simulink model "scanner_design_3d"  (R2023a)
settings: Solver=VariableStepAuto  StartTime=0.0  StopTime=10.0  RelTol=1e-3
settings Model: Creator=lenovo  LastModifiedBy=lenovo

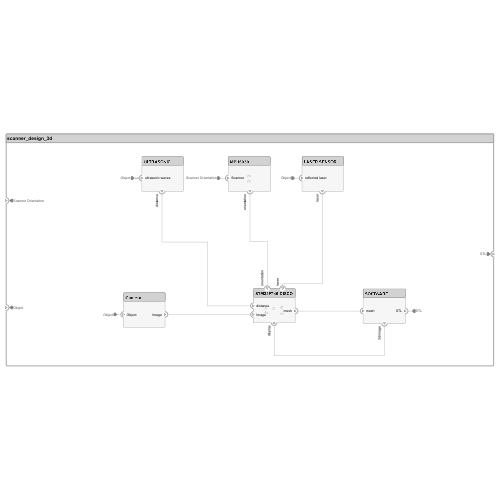
[thumbnail: Simulink's stored preview of the top-level diagram]
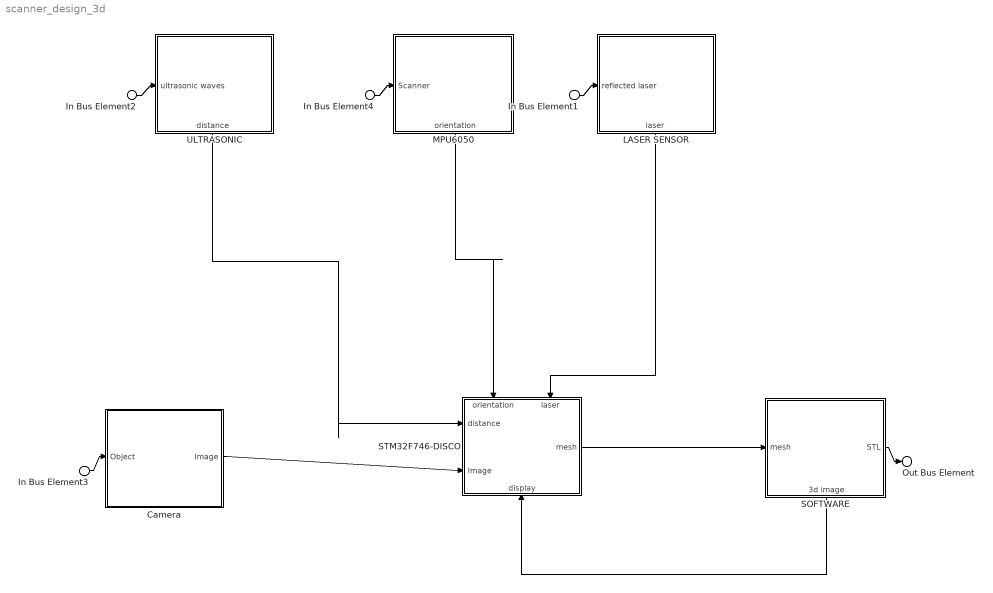
== system scanner_design_3d ==
  In Bus Element4 : Inport  PortName=Scanner Orientation
  In Bus Element1 : Inport  Port=2  PortName=Object
  In Bus Element3 : Inport  Port=2  PortName=Object
  In Bus Element2 : Inport  Port=2  PortName=Object
  Camera : Subsystem
      settings: PortSchema="{\"entries\":[{\"content\":{\"headerSize\":26,\"margin\":15,\"minimumSpacing\":25,\"sides\":[{\"content\":{\"connectorIds\":[\"In1\"]},\"type\":\"ConnectorPlacement.EquallySpacedRectSide\",\"uuid\":\"2eee4fd0-a715-4275-a226-480a0d6abb5e\"},{\"content\":{\"connectorIds\":[\"Out1\"],\"side\":\"RIGHT\"},\"type\":\"ConnectorPlacement.EquallySpacedRectSide\",\"uuid\":\"cdef6956-26e3-4994-be7c-9f37706eab71\"},{\"content\":{\"side\":\"TOP\"},\"type\":\"ConnectorPlacement.EquallySpacedRectSide\",\"uuid\":\"d49d9082-8e39-4dea-9a4e-805e3e59c1db\"}]},\"type\":\"ConnectorPlacement.EquallySpacedConnector\",\"uuid\":\"d2393f48-2e3c-4715-90d2-b77770385fe3\"}],\"packageUris\":[\"http://schema.mathworks.com/mf0/Connector/R2020b\"],\"version\":\"1.0\"}"
  LASER SENSOR : Subsystem
      settings: PortSchema="{\"entries\":[{\"content\":{\"headerSize\":26,\"margin\":15,\"minimumSpacing\":25,\"sides\":[{\"content\":{\"connectorIds\":[\"In1\"]},\"type\":\"ConnectorPlacement.EquallySpacedRectSide\",\"uuid\":\"2eee4fd0-a715-4275-a226-480a0d6abb5e\"},{\"content\":{\"side\":\"RIGHT\"},\"type\":\"ConnectorPlacement.EquallySpacedRectSide\",\"uuid\":\"cdef6956-26e3-4994-be7c-9f37706eab71\"},{\"content\":{\"side\":\"TOP\"},\"type\":\"ConnectorPlacement.EquallySpacedRectSide\",\"uuid\":\"d49d9082-8e39-4dea-9a4e-805e3e59c1db\"},{\"content\":{\"connectorIds\":[\"Out1\"],\"side\":\"BOTTOM\"},\"type\":\"ConnectorPlacement.EquallySpacedRectSide\",\"uuid\":\"d8085a13-85a2-42d5-92f1-ff20fd15cc84\"}]},\"type\":\"ConnectorPlacement.EquallySpacedConnector\",\"uuid\":\"d2393f48-2e3c-4715-90d2-b77770385fe3\"}],\"packageUris\":[\"http://schema.mathworks.com/mf0/Connector/R2020b\"],\"version\":\"1.0\"}"
  MPU6050 : Subsystem
      settings: PortSchema="{\"entries\":[{\"content\":{\"headerSize\":26,\"margin\":15,\"minimumSpacing\":25,\"sides\":[{\"content\":{\"connectorIds\":[\"In1\"]},\"type\":\"ConnectorPlacement.EquallySpacedRectSide\",\"uuid\":\"2eee4fd0-a715-4275-a226-480a0d6abb5e\"},{\"content\":{\"side\":\"RIGHT\"},\"type\":\"ConnectorPlacement.EquallySpacedRectSide\",\"uuid\":\"cdef6956-26e3-4994-be7c-9f37706eab71\"},{\"content\":{\"side\":\"TOP\"},\"type\":\"ConnectorPlacement.EquallySpacedRectSide\",\"uuid\":\"d49d9082-8e39-4dea-9a4e-805e3e59c1db\"},{\"content\":{\"connectorIds\":[\"Out1\"],\"side\":\"BOTTOM\"},\"type\":\"ConnectorPlacement.EquallySpacedRectSide\",\"uuid\":\"b078de67-0ec8-4653-9c4d-612ceac8148a\"}]},\"type\":\"ConnectorPlacement.EquallySpacedConnector\",\"uuid\":\"d2393f48-2e3c-4715-90d2-b77770385fe3\"}],\"packageUris\":[\"http://schema.mathworks.com/mf0/Connector/R2020b\"],\"version\":\"1.0\"}"
  SOFTWARE : Subsystem
      settings: PortSchema="{\"entries\":[{\"content\":{\"headerSize\":26,\"margin\":15,\"minimumSpacing\":25,\"sides\":[{\"content\":{\"connectorIds\":[\"In1\"]},\"type\":\"ConnectorPlacement.EquallySpacedRectSide\",\"uuid\":\"2eee4fd0-a715-4275-a226-480a0d6abb5e\"},{\"content\":{\"connectorIds\":[\"Out1\"],\"side\":\"RIGHT\"},\"type\":\"ConnectorPlacement.EquallySpacedRectSide\",\"uuid\":\"cdef6956-26e3-4994-be7c-9f37706eab71\"},{\"content\":{\"side\":\"TOP\"},\"type\":\"ConnectorPlacement.EquallySpacedRectSide\",\"uuid\":\"d49d9082-8e39-4dea-9a4e-805e3e59c1db\"},{\"content\":{\"connectorIds\":[\"Out2\"],\"side\":\"BOTTOM\"},\"type\":\"ConnectorPlacement.EquallySpacedRectSide\",\"uuid\":\"0b6c6432-b892-45d8-8b41-6b664d115c4f\"}]},\"type\":\"ConnectorPlacement.EquallySpacedConnector\",\"uuid\":\"d2393f48-2e3c-4715-90d2-b77770385fe3\"}],\"packageUris\":[\"http://schema.mathworks.com/mf0/Connector/R2020b\"],\"version\":\"1.0\"}"
  STM32F746-DISCO : Subsystem
      settings: PortSchema="{\"entries\":[{\"content\":{\"headerSize\":26,\"margin\":15,\"minimumSpacing\":25,\"sides\":[{\"content\":{\"connectorIds\":[\"In3\",\"In2\"]},\"type\":\"ConnectorPlacement.EquallySpacedRectSide\",\"uuid\":\"2eee4fd0-a715-4275-a226-480a0d6abb5e\"},{\"content\":{\"connectorIds\":[\"Out1\"],\"side\":\"RIGHT\"},\"type\":\"ConnectorPlacement.EquallySpacedRectSide\",\"uuid\":\"cdef6956-26e3-4994-be7c-9f37706eab71\"},{\"content\":{\"connectorIds\":[\"In4\",\"In5\"],\"side\":\"TOP\"},\"type\":\"ConnectorPlacement.EquallySpacedRectSide\",\"uuid\":\"d49d9082-8e39-4dea-9a4e-805e3e59c1db\"},{\"content\":{\"connectorIds\":[\"In1\"],\"side\":\"BOTTOM\"},\"type\":\"ConnectorPlacement.EquallySpacedRectSide\",\"uuid\":\"f1ce8cd9-933c-4617-8e31-b493098c4f66\"}]},\"type\":\"ConnectorPlacement.EquallySpacedConnector\",\"uuid\":\"d2393f48-2e3c-4715-90d2-b77770385fe3\"}],\"packageUris\":[\"http://schema.mathworks.com/mf0/Connector/R2020b\"],\"version\":\"1.0\"}"
  ULTRASONIC : Subsystem
      settings: PortSchema="{\"entries\":[{\"content\":{\"headerSize\":26,\"margin\":15,\"minimumSpacing\":25,\"sides\":[{\"content\":{\"connectorIds\":[\"In1\"]},\"type\":\"ConnectorPlacement.EquallySpacedRectSide\",\"uuid\":\"2eee4fd0-a715-4275-a226-480a0d6abb5e\"},{\"content\":{\"side\":\"RIGHT\"},\"type\":\"ConnectorPlacement.EquallySpacedRectSide\",\"uuid\":\"cdef6956-26e3-4994-be7c-9f37706eab71\"},{\"content\":{\"side\":\"TOP\"},\"type\":\"ConnectorPlacement.EquallySpacedRectSide\",\"uuid\":\"d49d9082-8e39-4dea-9a4e-805e3e59c1db\"},{\"content\":{\"connectorIds\":[\"Out1\"],\"side\":\"BOTTOM\"},\"type\":\"ConnectorPlacement.EquallySpacedRectSide\",\"uuid\":\"2292e6e7-3722-4da3-a436-d6cbf2db6c09\"}]},\"type\":\"ConnectorPlacement.EquallySpacedConnector\",\"uuid\":\"d2393f48-2e3c-4715-90d2-b77770385fe3\"}],\"packageUris\":[\"http://schema.mathworks.com/mf0/Connector/R2020b\"],\"version\":\"1.0\"}"
  Out Bus Element : Outport  PortName=STL
  wires:
  MPU6050/1(orientation) -> STM32F746-DISCO/4(orientation)
  LASER SENSOR/1(laser) -> STM32F746-DISCO/5(laser)
  STM32F746-DISCO/1(mesh) -> SOFTWARE/1(mesh)
  ULTRASONIC/1(distance) -> STM32F746-DISCO/3(distance)
  SOFTWARE/2(3d image) -> STM32F746-DISCO/1(display)
  SOFTWARE/1(STL) -> Out Bus Element/1
  In Bus Element1/1 -> LASER SENSOR/1(reflected laser)
  In Bus Element3/1 -> Camera/1(Object)
  Camera/1(Image) -> STM32F746-DISCO/2(Image)
  In Bus Element4/1 -> MPU6050/1(Scanner)
  In Bus Element2/1 -> ULTRASONIC/1(ultrasonic waves)

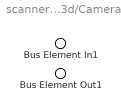
== system scanner_design_3d/Camera ==
  Bus Element In1 : Inport  PortName=Object
  Bus Element Out1 : Outport  PortName=Image

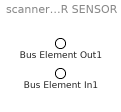
== system scanner_design_3d/LASER SENSOR ==
  Bus Element In1 : Inport  PortName=reflected laser
  Bus Element Out1 : Outport  PortName=laser

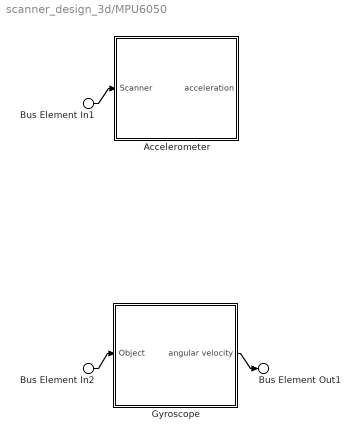
== system scanner_design_3d/MPU6050 ==
  Bus Element In1 : Inport  PortName=Scanner
  Bus Element In2 : Inport  PortName=Scanner
  Accelerometer : Subsystem
      settings: PortSchema="{\"entries\":[{\"content\":{\"headerSize\":26,\"margin\":15,\"minimumSpacing\":25,\"sides\":[{\"content\":{\"connectorIds\":[\"In1\"]},\"type\":\"ConnectorPlacement.EquallySpacedRectSide\",\"uuid\":\"2eee4fd0-a715-4275-a226-480a0d6abb5e\"},{\"content\":{\"connectorIds\":[\"Out1\"],\"side\":\"RIGHT\"},\"type\":\"ConnectorPlacement.EquallySpacedRectSide\",\"uuid\":\"cdef6956-26e3-4994-be7c-9f37706eab71\"},{\"content\":{\"side\":\"TOP\"},\"type\":\"ConnectorPlacement.EquallySpacedRectSide\",\"uuid\":\"d49d9082-8e39-4dea-9a4e-805e3e59c1db\"}]},\"type\":\"ConnectorPlacement.EquallySpacedConnector\",\"uuid\":\"d2393f48-2e3c-4715-90d2-b77770385fe3\"}],\"packageUris\":[\"http://schema.mathworks.com/mf0/Connector/R2020b\"],\"version\":\"1.0\"}"
  Gyroscope : Subsystem
      settings: PortSchema="{\"entries\":[{\"content\":{\"headerSize\":26,\"margin\":15,\"minimumSpacing\":25,\"sides\":[{\"content\":{\"connectorIds\":[\"In1\"]},\"type\":\"ConnectorPlacement.EquallySpacedRectSide\",\"uuid\":\"2eee4fd0-a715-4275-a226-480a0d6abb5e\"},{\"content\":{\"connectorIds\":[\"Out1\"],\"side\":\"RIGHT\"},\"type\":\"ConnectorPlacement.EquallySpacedRectSide\",\"uuid\":\"cdef6956-26e3-4994-be7c-9f37706eab71\"},{\"content\":{\"side\":\"TOP\"},\"type\":\"ConnectorPlacement.EquallySpacedRectSide\",\"uuid\":\"d49d9082-8e39-4dea-9a4e-805e3e59c1db\"}]},\"type\":\"ConnectorPlacement.EquallySpacedConnector\",\"uuid\":\"d2393f48-2e3c-4715-90d2-b77770385fe3\"}],\"packageUris\":[\"http://schema.mathworks.com/mf0/Connector/R2020b\"],\"version\":\"1.0\"}"
  Bus Element Out1 : Outport  PortName=orientation
  wires:
  Bus Element In1/1 -> Accelerometer/1(Scanner)
  Bus Element In2/1 -> Gyroscope/1(Object)
  Gyroscope/1(angular velocity) -> Bus Element Out1/1

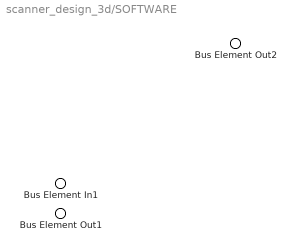
== system scanner_design_3d/SOFTWARE ==
  Bus Element In1 : Inport  PortName=mesh
  Bus Element Out2 : Outport  PortName=STL
  Bus Element Out1 : Outport  Port=2  PortName=3d image

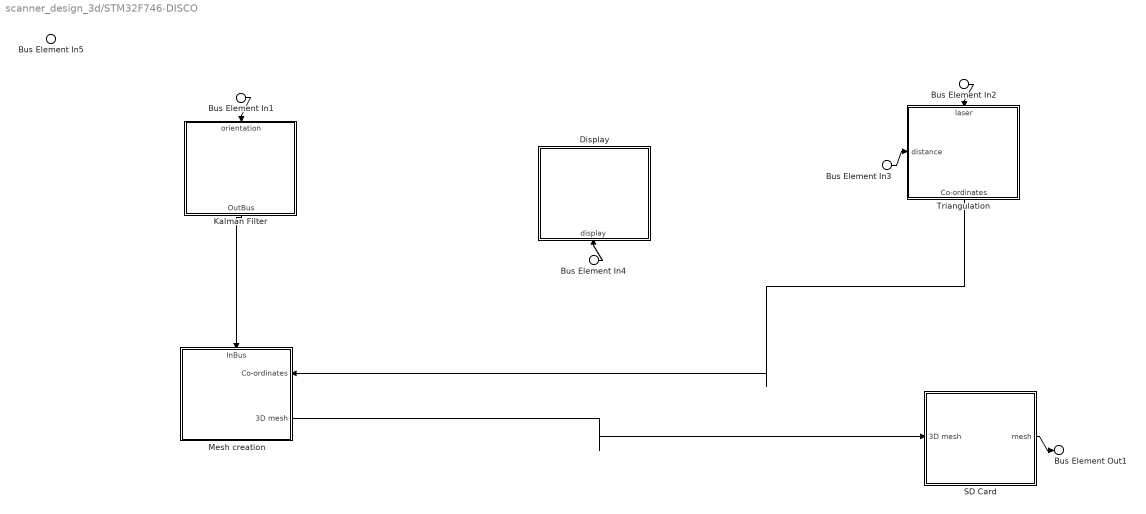
== system scanner_design_3d/STM32F746-DISCO ==
  Bus Element In4 : Inport  PortName=display
  Bus Element In5 : Inport  Port=2  PortName=Image
  Bus Element In3 : Inport  Port=3  PortName=distance
  Bus Element In1 : Inport  Port=4  PortName=orientation
  Bus Element In2 : Inport  Port=5  PortName=laser
  Display : Subsystem
      settings: PortSchema="{\"entries\":[{\"content\":{\"headerSize\":26,\"margin\":15,\"minimumSpacing\":25,\"sides\":[{\"content\":{},\"type\":\"ConnectorPlacement.EquallySpacedRectSide\",\"uuid\":\"2eee4fd0-a715-4275-a226-480a0d6abb5e\"},{\"content\":{\"side\":\"RIGHT\"},\"type\":\"ConnectorPlacement.EquallySpacedRectSide\",\"uuid\":\"cdef6956-26e3-4994-be7c-9f37706eab71\"},{\"content\":{\"side\":\"TOP\"},\"type\":\"ConnectorPlacement.EquallySpacedRectSide\",\"uuid\":\"d49d9082-8e39-4dea-9a4e-805e3e59c1db\"},{\"content\":{\"connectorIds\":[\"In1\"],\"side\":\"BOTTOM\"},\"type\":\"ConnectorPlacement.EquallySpacedRectSide\",\"uuid\":\"105528ff-cbad-49ac-870a-815d8629b1de\"}]},\"type\":\"ConnectorPlacement.EquallySpacedConnector\",\"uuid\":\"d2393f48-2e3c-4715-90d2-b77770385fe3\"}],\"packageUris\":[\"http://schema.mathworks.com/mf0/Connector/R2020b\"],\"version\":\"1.0\"}"
  Kalman Filter : Subsystem
      settings: PortSchema="{\"entries\":[{\"content\":{\"headerSize\":26,\"margin\":15,\"minimumSpacing\":25,\"sides\":[{\"content\":{},\"type\":\"ConnectorPlacement.EquallySpacedRectSide\",\"uuid\":\"2eee4fd0-a715-4275-a226-480a0d6abb5e\"},{\"content\":{\"side\":\"RIGHT\"},\"type\":\"ConnectorPlacement.EquallySpacedRectSide\",\"uuid\":\"cdef6956-26e3-4994-be7c-9f37706eab71\"},{\"content\":{\"connectorIds\":[\"In1\"],\"side\":\"TOP\"},\"type\":\"ConnectorPlacement.EquallySpacedRectSide\",\"uuid\":\"d49d9082-8e39-4dea-9a4e-805e3e59c1db\"},{\"content\":{\"connectorIds\":[\"Out1\"],\"side\":\"BOTTOM\"},\"type\":\"ConnectorPlacement.EquallySpacedRectSide\",\"uuid\":\"56c996cd-020d-4f5b-ad8e-252d506fa5fa\"}]},\"type\":\"ConnectorPlacement.EquallySpacedConnector\",\"uuid\":\"d2393f48-2e3c-4715-90d2-b77770385fe3\"}],\"packageUris\":[\"http://schema.mathworks.com/mf0/Connector/R2020b\"],\"version\":\"1.0\"}"
  Mesh creation : Subsystem
      settings: PortSchema="{\"entries\":[{\"content\":{\"headerSize\":26,\"margin\":15,\"minimumSpacing\":25,\"sides\":[{\"content\":{},\"type\":\"ConnectorPlacement.EquallySpacedRectSide\",\"uuid\":\"2eee4fd0-a715-4275-a226-480a0d6abb5e\"},{\"content\":{\"connectorIds\":[\"In1\",\"Out1\"],\"side\":\"RIGHT\"},\"type\":\"ConnectorPlacement.EquallySpacedRectSide\",\"uuid\":\"cdef6956-26e3-4994-be7c-9f37706eab71\"},{\"content\":{\"connectorIds\":[\"In2\"],\"side\":\"TOP\"},\"type\":\"ConnectorPlacement.EquallySpacedRectSide\",\"uuid\":\"d49d9082-8e39-4dea-9a4e-805e3e59c1db\"}]},\"type\":\"ConnectorPlacement.EquallySpacedConnector\",\"uuid\":\"d2393f48-2e3c-4715-90d2-b77770385fe3\"}],\"packageUris\":[\"http://schema.mathworks.com/mf0/Connector/R2020b\"],\"version\":\"1.0\"}"
  SD Card : Subsystem
      settings: PortSchema="{\"entries\":[{\"content\":{\"headerSize\":26,\"margin\":15,\"minimumSpacing\":25,\"sides\":[{\"content\":{\"connectorIds\":[\"In1\"]},\"type\":\"ConnectorPlacement.EquallySpacedRectSide\",\"uuid\":\"2eee4fd0-a715-4275-a226-480a0d6abb5e\"},{\"content\":{\"connectorIds\":[\"Out1\"],\"side\":\"RIGHT\"},\"type\":\"ConnectorPlacement.EquallySpacedRectSide\",\"uuid\":\"cdef6956-26e3-4994-be7c-9f37706eab71\"},{\"content\":{\"side\":\"TOP\"},\"type\":\"ConnectorPlacement.EquallySpacedRectSide\",\"uuid\":\"d49d9082-8e39-4dea-9a4e-805e3e59c1db\"}]},\"type\":\"ConnectorPlacement.EquallySpacedConnector\",\"uuid\":\"d2393f48-2e3c-4715-90d2-b77770385fe3\"}],\"packageUris\":[\"http://schema.mathworks.com/mf0/Connector/R2020b\"],\"version\":\"1.0\"}"
  Triangulation : Subsystem
      settings: PortSchema="{\"entries\":[{\"content\":{\"headerSize\":26,\"margin\":15,\"minimumSpacing\":25,\"sides\":[{\"content\":{\"connectorIds\":[\"In2\"]},\"type\":\"ConnectorPlacement.EquallySpacedRectSide\",\"uuid\":\"2eee4fd0-a715-4275-a226-480a0d6abb5e\"},{\"content\":{\"side\":\"RIGHT\"},\"type\":\"ConnectorPlacement.EquallySpacedRectSide\",\"uuid\":\"cdef6956-26e3-4994-be7c-9f37706eab71\"},{\"content\":{\"connectorIds\":[\"In1\"],\"side\":\"TOP\"},\"type\":\"ConnectorPlacement.EquallySpacedRectSide\",\"uuid\":\"d49d9082-8e39-4dea-9a4e-805e3e59c1db\"},{\"content\":{\"connectorIds\":[\"Out1\"],\"side\":\"BOTTOM\"},\"type\":\"ConnectorPlacement.EquallySpacedRectSide\",\"uuid\":\"b3e2cf29-4f6d-4746-8d0c-edd739d1bc30\"}]},\"type\":\"ConnectorPlacement.EquallySpacedConnector\",\"uuid\":\"d2393f48-2e3c-4715-90d2-b77770385fe3\"}],\"packageUris\":[\"http://schema.mathworks.com/mf0/Connector/R2020b\"],\"version\":\"1.0\"}"
  Bus Element Out1 : Outport  PortName=mesh
  wires:
  Bus Element In1/1 -> Kalman Filter/1(orientation)
  Kalman Filter/1(OutBus) -> Mesh creation/2(InBus)
  Mesh creation/1(3D mesh) -> SD Card/1(3D mesh)
  Bus Element In3/1 -> Triangulation/2(distance)
  Bus Element In2/1 -> Triangulation/1(laser)
  SD Card/1(mesh) -> Bus Element Out1/1
  Triangulation/1(Co-ordinates) -> Mesh creation/1(Co-ordinates)
  Bus Element In4/1 -> Display/1(display)

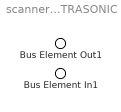
== system scanner_design_3d/ULTRASONIC ==
  Bus Element In1 : Inport  PortName=ultrasonic waves
  Bus Element Out1 : Outport  PortName=distance

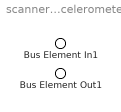
== system scanner_design_3d/MPU6050/Accelerometer ==
  Bus Element In1 : Inport  PortName=Scanner
  Bus Element Out1 : Outport  PortName=acceleration

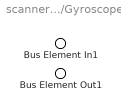
== system scanner_design_3d/MPU6050/Gyroscope ==
  Bus Element In1 : Inport  PortName=Object
  Bus Element Out1 : Outport  PortName=angular velocity

== system scanner_design_3d/STM32F746-DISCO/Display ==
  Bus Element In1 : Inport  PortName=display

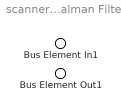
== system scanner_design_3d/STM32F746-DISCO/Kalman Filter ==
  Bus Element In1 : Inport  PortName=orientation
  Bus Element Out1 : Outport  PortName=OutBus

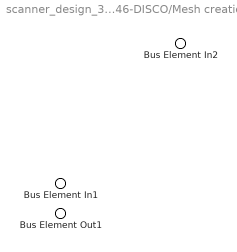
== system scanner_design_3d/STM32F746-DISCO/Mesh creation ==
  Bus Element In2 : Inport  PortName=Co-ordinates
  Bus Element In1 : Inport  Port=2  PortName=InBus
  Bus Element Out1 : Outport  PortName=3D mesh

== system scanner_design_3d/STM32F746-DISCO/SD Card ==
  Bus Element In1 : Inport  PortName=3D mesh
  Bus Element Out1 : Outport  PortName=mesh

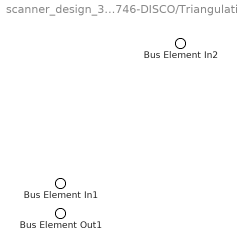
== system scanner_design_3d/STM32F746-DISCO/Triangulation ==
  Bus Element In2 : Inport  PortName=laser
  Bus Element In1 : Inport  Port=2  PortName=distance
  Bus Element Out1 : Outport  PortName=Co-ordinates
